simulink model "b1"  (R2020a)
settings: Solver=VariableStepAuto  StartTime=0.0  StopTime=10.0  RelTol=1e-3
settings Model: Creator=Erfan  LastModifiedBy=Erfan

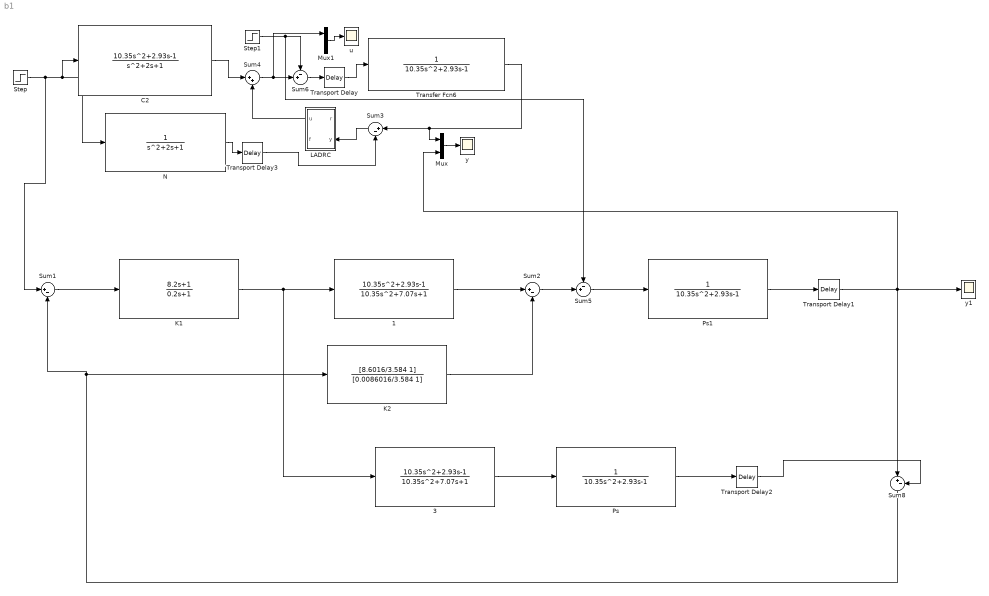
== system b1 ==
  1 : TransferFcn  Numerator=[10.35 2.93 -1]  Denominator=[10.35 7.07 1]
  3 : TransferFcn  Numerator=[10.35 2.93 -1]  Denominator=[10.35 7.07 1]
  C2 : TransferFcn  Numerator=[10.35 2.93 -1]
  K1 : TransferFcn  Numerator=[8.2 1]  Denominator=[0.2 1]
  K2 : TransferFcn  Numerator=[8.6016/3.584 1]  Denominator=[0.0086016/3.584 1]
  LADRC : Subsystem  mask{n=3, b0=1, Ko=[9406.895 998.3894 56.6806 1], Lo=[4.1063 17.5144 10.875 1.6927]'}
      mask prompts: n "order"; b0 "high-frequency gain"; Ko "feedback gain"; Lo "observer gain"
  Mux : Mux  Inputs=2
  Mux1 : Mux  Inputs=2
  N : TransferFcn  Numerator=1
  Ps : TransferFcn  Numerator=1  Denominator=[10.35 2.93 -1]
  Ps1 : TransferFcn  Numerator=1  Denominator=[10.35 2.93 -1]
  Step : Step  Time=0  SampleTime=0
  Step1 : Step  Time=20  SampleTime=0
  Sum{1..3,8} (4 alike) : Sum  Inputs=|+-  SaturateOnIntegerOverflow=on
  Sum4 : Sum  Inputs=|++  SaturateOnIntegerOverflow=on
  Sum5 : Sum  Inputs=-+|  SaturateOnIntegerOverflow=on
  Sum6 : Sum  Inputs=-+|  InputSameDT=on  SaturateOnIntegerOverflow=on  OutDataTypeStr=Inherit: Same as first input
  Transfer Fcn6 : TransferFcn  Numerator=1  Denominator=[10.35 2.93 -1]
  Transport Delay{,1..3} (4 alike) : TransportDelay  DelayTime=0.939
  u : Scope
  y : Scope
  y1 : Scope
  wires:
  LADRC/1(u) -> Sum4/2
  Ps/1 -> Transport Delay2/1
  Step/1 -> Sum1/1, N/1, C2/1
  Sum3/1 -> LADRC/2(y)
  Step1/1 -> Sum5/1, Sum6/1
  Sum1/1 -> K1/1
  Sum5/1 -> Ps1/1
  K2/1 -> Sum2/2
  3/1 -> Ps/1
  Transport Delay/1 -> Transfer Fcn6/1
  Sum8/1 -> K2/1, Sum1/2
  Mux1/1 -> u/1
  Transport Delay2/1 -> Sum8/2
  Transfer Fcn6/1 -> Mux/1, Sum3/1
  Ps1/1 -> Transport Delay1/1
  Transport Delay1/1 -> Mux/2, y1/1, Sum8/1
  C2/1 -> Sum4/1
  Sum2/1 -> Sum5/2
  Sum4/1 -> Mux1/1, Sum6/2
  Sum6/1 -> Transport Delay/1
  1/1 -> Sum2/1
  K1/1 -> 3/1, 1/1
  N/1 -> Transport Delay3/1
  Transport Delay3/1 -> Sum3/2
  Mux/1 -> y/1

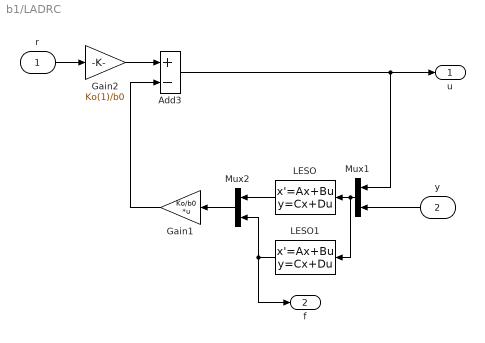
== system b1/LADRC ==
  r : Inport
  y : Inport  Port=2
  Add3 : Sum  Inputs=+-
  Gain1 : Gain  Gain=Ko/b0  Multiplication=Matrix(K*u)
  Gain2 : Gain  Gain=Ko(1)/b0
  LESO : StateSpace  A=[zeros(n,1) eye(n,n);zeros(1,n+1)]-Lo*[1 zeros(1,n)]  B=[[zeros(n-1,1);b0;0] Lo]  C=[eye(n,n) zeros(n,1)]  D=zeros(n,2)  InitialCondition=0
  LESO1 : StateSpace  A=[zeros(n,1) eye(n,n);zeros(1,n+1)]-Lo*[1 zeros(1,n)]  B=[[zeros(n-1,1);b0;0] Lo]  C=[zeros(1,n) 1]  D=[0 0]  InitialCondition=0
  Mux1 : Mux  Inputs=2
  Mux2 : Mux  Inputs=2
  u : Outport
  f : Outport  Port=2
  wires:
  Gain1/1 -> Add3/2
  LESO1/1 -> Mux2/2, f/1
  Mux2/1 -> Gain1/1
  LESO/1 -> Mux2/1
  r/1 -> Gain2/1
  Mux1/1 -> LESO/1, LESO1/1
  y/1 -> Mux1/2
  Add3/1 -> Mux1/1, u/1
  Gain2/1 -> Add3/1
